simulink model "Example_8_4b"  (R2014a)
settings: Solver=FixedStepDiscrete  SolverMode=SingleTasking  StartTime=0.0  StopTime=inf  RelTol=1e-3
libraries: simulink x2
settings Model: Creator=Lee Edwards  LastModifiedBy=Lee
settings DataIOCC: SignalLoggingSaveFormat=ModelDataLogs  SaveOutput=off  SignalLogging=off  SaveTime=off
settings OptimizationCC: ExpressionDepthLimit=2147483647
settings DebuggingCC: AlgebraicLoopMsg=error  UnderspecifiedInitializationDetection=Classic  SingleTaskRateTransMsg=error  FcnCallInpInsideContextMsg=UseLocalSettings  StateNameClashWarn=warning  StrictBusMsg=Warning
settings GRTTargetCC: CombineOutputUpdateFcns=off  GRTInterface=on

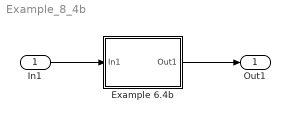
== system Example_8_4b ==
  In1 : Inport
  Example 6.4b : Subsystem
  Out1 : Outport
  wires:
  In1/1 -> Example 6.4b/1(In1)
  Example 6.4b/1(Out1) -> Out1/1

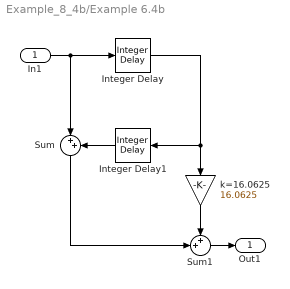
== system Example_8_4b/Example 6.4b ==
  In1 : Inport
  Integer Delay : simulink/Discrete/Integer Delay  NumDelays=4  vinit=0.0  samptime=-1
  Integer Delay1 : simulink/Discrete/Integer Delay  NumDelays=4  vinit=0.0  samptime=-1
  Sum : Sum  Inputs=|++
  Sum1 : Sum  Inputs=++|
  k=16.0625 : Gain  Gain=16.0625
  Out1 : Outport
  wires:
  In1/1 -> Integer Delay/1, Sum/1
  Integer Delay/1 -> Integer Delay1/1, k=16.0625/1
  Integer Delay1/1 -> Sum/2
  Sum/1 -> Sum1/2
  k=16.0625/1 -> Sum1/1
  Sum1/1 -> Out1/1
